simulink model "IMU_Simulation"  (Simulink 7.9)
settings: Solver=FixedStepDiscrete  StartTime=0.0  StopTime=25  FixedStep=.001  RelTol=1e-3
PreLoadFcn:
  | Script_Kalman
values from neighbouring files (symbols this model uses):
  Az = [1 -Ts ;0 1]    [Script_Kalman.m]
  Kz = 1e-3*[.4 ; -.04]    [Script_Kalman.m]
  Ts = .001    (= 0.001)    [Script_Kalman.m]
undefined symbols (not defined in the file or in its folder): dend, DiscIntNeverNeededParam, gaind, numd, polesd, zerosd
libraries: simulink x38
(part 2 of 2)

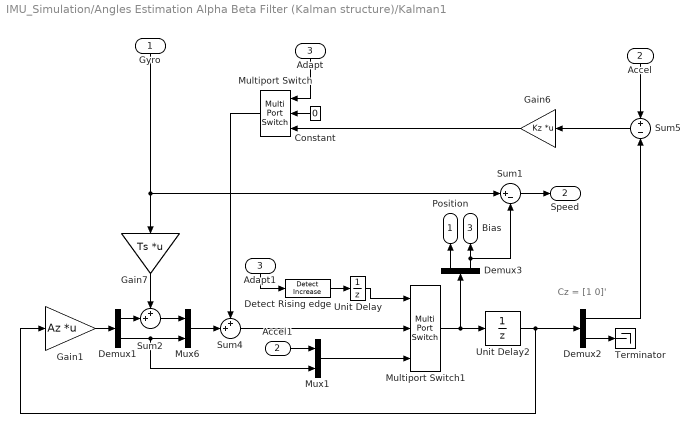
== system IMU_Simulation/Angles Estimation Alpha Beta Filter (Kalman structure)/Kalman1 ==
  note: Cz = [1 0]'
  Gyro : Inport
  Accel : Inport  Port=2
  Adapt : Inport  Port=3
  Accel1 : InportShadow  Port=2
  Adapt1 : InportShadow  Port=3
  Constant : Constant  Value=0
  Demux1 : Demux  Outputs=2
  Demux2 : Demux  Outputs=2
  Demux3 : Demux  Outputs=2
  Detect Rising edge : simulink/Logic and Bit Operations/Detect Increase  vinit=0  InputProcessing=Inherited  OutDataTypeStr=uint8
  Gain1 : Gain  Gain=Az  Multiplication=Matrix(K*u)
  Gain6 : Gain  Gain=Kz  Multiplication=Matrix(K*u)
  Gain7 : Gain  Gain=Ts  Multiplication=Matrix(K*u)
  Multiport Switch : MultiPortSwitch  DataPortOrder=Zero-based contiguous  Inputs=2  zeroidx=on
  Multiport Switch1 : MultiPortSwitch  DataPortOrder=Zero-based contiguous  Inputs=2  zeroidx=on
  Mux1 : Mux  Inputs=2
  Mux6 : Mux  Inputs=2
  Sum1 : Sum  Inputs=|+-
  Sum2 : Sum  Inputs=++|
  Sum4 : Sum  Inputs=++|
  Sum5 : Sum  Inputs=+-
  Terminator : Terminator
  Unit Delay : UnitDelay  SampleTime=-1
  Unit Delay2 : UnitDelay  SampleTime=-1
  Position : Outport
  Speed : Outport  Port=2
  Bias : Outport  Port=3
  wires:
  Sum1/1 -> Speed/1
  Demux3/2 -> Sum1/2, Bias/1
  Demux3/1 -> Position/1
  Unit Delay2/1 -> Gain1/1, Demux2/1
  Unit Delay/1 -> Multiport Switch1/1
  Gyro/1 -> Sum1/1, Gain7/1
  Accel/1 -> Sum5/1
  Gain7/1 -> Sum2/1
  Sum5/1 -> Gain6/1
  Mux6/1 -> Sum4/2
  Demux1/2 -> Mux6/2, Mux1/2
  Sum2/1 -> Mux6/1
  Demux1/1 -> Sum2/2
  Gain1/1 -> Demux1/1
  Demux2/1 -> Sum5/2
  Multiport Switch/1 -> Sum4/1
  Adapt/1 -> Multiport Switch/1
  Gain6/1 -> Multiport Switch/3
  Constant/1 -> Multiport Switch/2
  Detect Rising edge/1 -> Unit Delay/1
  Multiport Switch1/1 -> Demux3/1, Unit Delay2/1
  Sum4/1 -> Multiport Switch1/2
  Adapt1/1 -> Detect Rising edge/1
  Accel1/1 -> Mux1/1
  Mux1/1 -> Multiport Switch1/3
  Demux2/2 -> Terminator/1

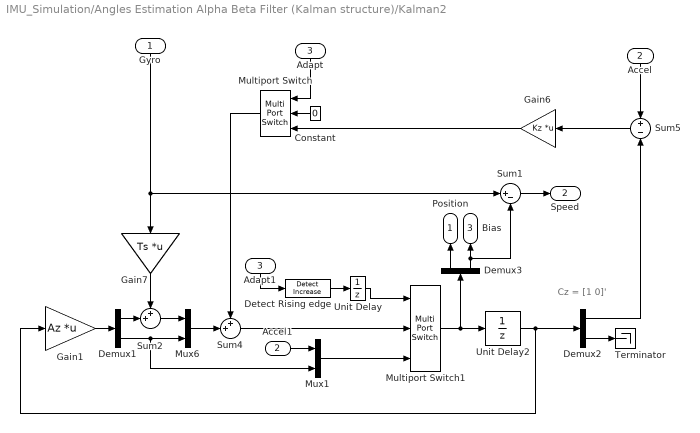
== system IMU_Simulation/Angles Estimation Alpha Beta Filter (Kalman structure)/Kalman2 ==
  note: Cz = [1 0]'
  Gyro : Inport
  Accel : Inport  Port=2
  Adapt : Inport  Port=3
  Accel1 : InportShadow  Port=2
  Adapt1 : InportShadow  Port=3
  Constant : Constant  Value=0
  Demux1 : Demux  Outputs=2
  Demux2 : Demux  Outputs=2
  Demux3 : Demux  Outputs=2
  Detect Rising edge : simulink/Logic and Bit Operations/Detect Increase  vinit=0  InputProcessing=Inherited  OutDataTypeStr=uint8
  Gain1 : Gain  Gain=Az  Multiplication=Matrix(K*u)
  Gain6 : Gain  Gain=Kz  Multiplication=Matrix(K*u)
  Gain7 : Gain  Gain=Ts  Multiplication=Matrix(K*u)
  Multiport Switch : MultiPortSwitch  DataPortOrder=Zero-based contiguous  Inputs=2  zeroidx=on
  Multiport Switch1 : MultiPortSwitch  DataPortOrder=Zero-based contiguous  Inputs=2  zeroidx=on
  Mux1 : Mux  Inputs=2
  Mux6 : Mux  Inputs=2
  Sum1 : Sum  Inputs=|+-
  Sum2 : Sum  Inputs=++|
  Sum4 : Sum  Inputs=++|
  Sum5 : Sum  Inputs=+-
  Terminator : Terminator
  Unit Delay : UnitDelay  SampleTime=-1
  Unit Delay2 : UnitDelay  SampleTime=-1
  Position : Outport
  Speed : Outport  Port=2
  Bias : Outport  Port=3
  wires:
  Demux2/2 -> Terminator/1
  Mux1/1 -> Multiport Switch1/3
  Accel1/1 -> Mux1/1
  Adapt1/1 -> Detect Rising edge/1
  Sum4/1 -> Multiport Switch1/2
  Multiport Switch1/1 -> Unit Delay2/1, Demux3/1
  Detect Rising edge/1 -> Unit Delay/1
  Constant/1 -> Multiport Switch/2
  Gain6/1 -> Multiport Switch/3
  Adapt/1 -> Multiport Switch/1
  Multiport Switch/1 -> Sum4/1
  Demux2/1 -> Sum5/2
  Gain1/1 -> Demux1/1
  Demux1/1 -> Sum2/2
  Sum2/1 -> Mux6/1
  Demux1/2 -> Mux1/2, Mux6/2
  Mux6/1 -> Sum4/2
  Sum5/1 -> Gain6/1
  Gain7/1 -> Sum2/1
  Accel/1 -> Sum5/1
  Gyro/1 -> Gain7/1, Sum1/1
  Unit Delay/1 -> Multiport Switch1/1
  Unit Delay2/1 -> Demux2/1, Gain1/1
  Demux3/1 -> Position/1
  Demux3/2 -> Bias/1, Sum1/2
  Sum1/1 -> Speed/1

== system IMU_Simulation/Angles Estimation Alpha Beta Filter (Kalman structure)/Norm L1 ==
  Accel Y : Inport
  Accel Z : Inport  Port=2
  Accel X : Inport  Port=3
  Abs : Abs
  Abs1 : Abs
  Abs2 : Abs
  Sum1 : Sum
  Sum3 : Sum
  abs(Y)+abs(Z) : Outport
  abs(X)+abs(Z) : Outport  Port=2
  wires:
  Abs/1 -> Sum3/1
  Abs1/1 -> Sum1/1, Sum3/2
  Accel Y/1 -> Abs/1
  Accel Z/1 -> Abs1/1
  Sum3/1 -> abs(Y)+abs(Z)/1
  Abs2/1 -> Sum1/2
  Accel X/1 -> Abs2/1
  Sum1/1 -> abs(X)+abs(Z)/1

== system IMU_Simulation/Angles Estimation Alpha Beta Filter (Kalman structure)/Simplified Kalman for publi ==
  note: Cz = [1 0]'
  Gyro : Inport
  Accel : Inport  Port=2
  Demux1 : Demux  Outputs=2
  Demux2 : Demux  Outputs=2
  Gain1 : Gain  Gain=Az  Multiplication=Matrix(K*u)
  Gain6 : Gain  Gain=Kz  Multiplication=Matrix(K*u)
  Gain7 : Gain  Gain=Ts  Multiplication=Matrix(K*u)
  Mux6 : Mux  Inputs=2
  Sum2 : Sum  Inputs=++|
  Sum4 : Sum  Inputs=++|
  Sum5 : Sum  Inputs=+-
  Terminator : Terminator
  Unit Delay2 : UnitDelay  SampleTime=-1
  Angle Estimation : Outport
  wires:
  Demux2/2 -> Terminator/1
  Sum4/1 -> Unit Delay2/1
  Demux2/1 -> Sum5/2, Angle Estimation/1
  Gain1/1 -> Demux1/1
  Demux1/1 -> Sum2/2
  Sum2/1 -> Mux6/1  "Angle Estimation"
  Demux1/2 -> Mux6/2  "Gyro Bias"
  Mux6/1 -> Sum4/2
  Sum5/1 -> Gain6/1
  Gain7/1 -> Sum2/1
  Accel/1 -> Sum5/1
  Gyro/1 -> Gain7/1
  Unit Delay2/1 -> Demux2/1, Gain1/1
  Gain6/1 -> Sum4/1

== system IMU_Simulation/Angles Estimation Alpha Beta Filter (Kalman structure)/Unwrap1 ==
  Estimated Angle : Inport
  Compare To Constant : simulink/Logic and Bit Operations/Compare To Constant  relop=>  const=180  OutDataTypeStr=uint8  ZeroCross=off
  Compare To Constant1 : simulink/Logic and Bit Operations/Compare To Constant  relop=<  const=-180  OutDataTypeStr=uint8  ZeroCross=off
  Compare To Zero : simulink/Logic and Bit Operations/Compare To Zero  relop=~=  OutDataTypeStr=uint8  ZeroCross=off
  Difference : simulink/Discrete/Difference  ICPrevInput=0.0  InputProcessing=Inherited  OutMin=[]  OutMax=[]  OutDataType=sfix(16)  OutScaling=2^-10  DoSatur=off
  Discrete-Time Integrator : DiscreteIntegrator  gainval=1000  SampleTime=-1  ICPrevOutput=DiscIntNeverNeededParam  ICPrevScaledInput=DiscIntNeverNeededParam
  Logical Operator : Logic  Operator=NOR  AllPortsSameDT=off  OutDataTypeStr=boolean
  Lookup Table : Lookup  InputValues=[-500 -195 195]  Table=[+360 0 -360]  LookUpMeth=Use Input Below
  Merge : Merge  Inputs=3
  Sum2 : Sum
  unwrap : Subsystem  TreatAsAtomicUnit=on
  unwrap1 : Subsystem  TreatAsAtomicUnit=on
  unwrap2 : Subsystem  TreatAsAtomicUnit=on
  unwrap angle : Outport
  Wrap : Outport  Port=2
  wires:
  Compare To Zero/1 -> Wrap/1
  Lookup Table/1 -> Compare To Zero/1, Sum2/1
  Merge/1 -> Sum2/2
  Sum2/1 -> Discrete-Time Integrator/1
  Difference/1 -> Compare To Constant/1, unwrap/1(In1), Compare To Constant1/1, unwrap1/1(In1), unwrap2/1(In1)
  Compare To Constant/1 -> Logical Operator/1, unwrap/Enable
  Compare To Constant1/1 -> unwrap1/Enable, Logical Operator/2
  Logical Operator/1 -> unwrap2/Enable
  unwrap2/1(Out1) -> Merge/1
  unwrap/1(Out1) -> Merge/2
  unwrap1/1(Out1) -> Merge/3
  Estimated Angle/1 -> Difference/1
  Discrete-Time Integrator/1 -> Lookup Table/1, unwrap angle/1

== system IMU_Simulation/Angles Estimation Alpha Beta Filter (Kalman structure)/Unwrap2 ==
  Estimated Angle : Inport
  Compare To Constant : simulink/Logic and Bit Operations/Compare To Constant  relop=>  const=180  OutDataTypeStr=uint8  ZeroCross=off
  Compare To Constant1 : simulink/Logic and Bit Operations/Compare To Constant  relop=<  const=-180  OutDataTypeStr=uint8  ZeroCross=off
  Compare To Zero : simulink/Logic and Bit Operations/Compare To Zero  relop=~=  OutDataTypeStr=uint8  ZeroCross=off
  Difference : simulink/Discrete/Difference  ICPrevInput=0.0  InputProcessing=Inherited  OutMin=[]  OutMax=[]  OutDataType=sfix(16)  OutScaling=2^-10  DoSatur=off
  Discrete-Time Integrator : DiscreteIntegrator  gainval=1000  SampleTime=-1  ICPrevOutput=DiscIntNeverNeededParam  ICPrevScaledInput=DiscIntNeverNeededParam
  Logical Operator : Logic  Operator=NOR  AllPortsSameDT=off  OutDataTypeStr=boolean
  Lookup Table : Lookup  InputValues=[-500 -195 195]  Table=[+360 0 -360]  LookUpMeth=Use Input Below
  Merge : Merge  Inputs=3
  Sum2 : Sum
  unwrap : Subsystem  TreatAsAtomicUnit=on
  unwrap1 : Subsystem  TreatAsAtomicUnit=on
  unwrap2 : Subsystem  TreatAsAtomicUnit=on
  unwrap angle : Outport
  Wrap : Outport  Port=2
  wires:
  Discrete-Time Integrator/1 -> unwrap angle/1, Lookup Table/1
  Estimated Angle/1 -> Difference/1
  unwrap1/1(Out1) -> Merge/3
  unwrap/1(Out1) -> Merge/2
  unwrap2/1(Out1) -> Merge/1
  Logical Operator/1 -> unwrap2/Enable
  Compare To Constant1/1 -> Logical Operator/2, unwrap1/Enable
  Compare To Constant/1 -> unwrap/Enable, Logical Operator/1
  Difference/1 -> unwrap2/1(In1), unwrap1/1(In1), Compare To Constant1/1, unwrap/1(In1), Compare To Constant/1
  Sum2/1 -> Discrete-Time Integrator/1
  Merge/1 -> Sum2/2
  Lookup Table/1 -> Sum2/1, Compare To Zero/1
  Compare To Zero/1 -> Wrap/1

== system IMU_Simulation/Angle Estimation Complementary Filter Order 1/Unwrap1/unwrap ==
  In1 : Inport
  Enable : EnablePort
  Bias2 : Constant  Value=-360
  Sum2 : Sum
  Out1 : Outport
  wires:
  Bias2/1 -> Sum2/2
  Sum2/1 -> Out1/1
  In1/1 -> Sum2/1

== system IMU_Simulation/Angle Estimation Complementary Filter Order 1/Unwrap1/unwrap1 ==
  In1 : Inport
  Enable : EnablePort
  Bias2 : Constant  Value=360
  Sum2 : Sum
  Out1 : Outport
  wires:
  Sum2/1 -> Out1/1
  Bias2/1 -> Sum2/2
  In1/1 -> Sum2/1

== system IMU_Simulation/Angle Estimation Complementary Filter Order 1/Unwrap1/unwrap2 ==
  In1 : Inport
  Enable : EnablePort
  Out1 : Outport
  wires:
  In1/1 -> Out1/1

== system IMU_Simulation/Angle Estimation Complementary Filter Order 1/Unwrap2/unwrap ==
  In1 : Inport
  Enable : EnablePort
  Bias2 : Constant  Value=-360
  Sum2 : Sum
  Out1 : Outport
  wires:
  In1/1 -> Sum2/1
  Sum2/1 -> Out1/1
  Bias2/1 -> Sum2/2

== system IMU_Simulation/Angle Estimation Complementary Filter Order 1/Unwrap2/unwrap1 ==
  In1 : Inport
  Enable : EnablePort
  Bias2 : Constant  Value=360
  Sum2 : Sum
  Out1 : Outport
  wires:
  In1/1 -> Sum2/1
  Bias2/1 -> Sum2/2
  Sum2/1 -> Out1/1

== system IMU_Simulation/Angle Estimation Complementary Filter Order 1/Unwrap2/unwrap2 ==
  In1 : Inport
  Enable : EnablePort
  Out1 : Outport
  wires:
  In1/1 -> Out1/1

== system IMU_Simulation/Angle Estimation Complementary Filter Order 2/Unwrap1/unwrap ==
  In1 : Inport
  Enable : EnablePort
  Bias2 : Constant  Value=-360
  Sum2 : Sum
  Out1 : Outport
  wires:
  In1/1 -> Sum2/1
  Sum2/1 -> Out1/1
  Bias2/1 -> Sum2/2

== system IMU_Simulation/Angle Estimation Complementary Filter Order 2/Unwrap1/unwrap1 ==
  In1 : Inport
  Enable : EnablePort
  Bias2 : Constant  Value=360
  Sum2 : Sum
  Out1 : Outport
  wires:
  In1/1 -> Sum2/1
  Bias2/1 -> Sum2/2
  Sum2/1 -> Out1/1

== system IMU_Simulation/Angle Estimation Complementary Filter Order 2/Unwrap1/unwrap2 ==
  In1 : Inport
  Enable : EnablePort
  Out1 : Outport
  wires:
  In1/1 -> Out1/1

== system IMU_Simulation/Angle Estimation Complementary Filter Order 2/Unwrap2/unwrap ==
  In1 : Inport
  Enable : EnablePort
  Bias2 : Constant  Value=-360
  Sum2 : Sum
  Out1 : Outport
  wires:
  Bias2/1 -> Sum2/2
  Sum2/1 -> Out1/1
  In1/1 -> Sum2/1

== system IMU_Simulation/Angle Estimation Complementary Filter Order 2/Unwrap2/unwrap1 ==
  In1 : Inport
  Enable : EnablePort
  Bias2 : Constant  Value=360
  Sum2 : Sum
  Out1 : Outport
  wires:
  Sum2/1 -> Out1/1
  Bias2/1 -> Sum2/2
  In1/1 -> Sum2/1

== system IMU_Simulation/Angle Estimation Complementary Filter Order 2/Unwrap2/unwrap2 ==
  In1 : Inport
  Enable : EnablePort
  Out1 : Outport
  wires:
  In1/1 -> Out1/1

== system IMU_Simulation/Angles Estimation (Ref: Pisano 2005)/Pisano/Low Pass1 ==
  In1 : Inport
  Discrete Zero-Pole : DiscreteZeroPole  Zeros=zerosd  Poles=polesd  Gain=gaind  SampleTime=SampleTime
  Out1 : Outport
  wires:
  Discrete Zero-Pole/1 -> Out1/1
  In1/1 -> Discrete Zero-Pole/1

== system IMU_Simulation/Angles Estimation (Ref: Pisano 2005)/Pisano1/Low Pass1 ==
  In1 : Inport
  Discrete Zero-Pole : DiscreteZeroPole  Zeros=zerosd  Poles=polesd  Gain=gaind  SampleTime=SampleTime
  Out1 : Outport
  wires:
  In1/1 -> Discrete Zero-Pole/1
  Discrete Zero-Pole/1 -> Out1/1

== system IMU_Simulation/Angles Estimation (Ref: Pisano 2005)/Unwrap1/unwrap ==
  In1 : Inport
  Enable : EnablePort
  Bias2 : Constant  Value=-360
  Sum2 : Sum
  Out1 : Outport
  wires:
  Bias2/1 -> Sum2/2
  Sum2/1 -> Out1/1
  In1/1 -> Sum2/1

== system IMU_Simulation/Angles Estimation (Ref: Pisano 2005)/Unwrap1/unwrap1 ==
  In1 : Inport
  Enable : EnablePort
  Bias2 : Constant  Value=360
  Sum2 : Sum
  Out1 : Outport
  wires:
  Sum2/1 -> Out1/1
  Bias2/1 -> Sum2/2
  In1/1 -> Sum2/1

== system IMU_Simulation/Angles Estimation (Ref: Pisano 2005)/Unwrap1/unwrap2 ==
  In1 : Inport
  Enable : EnablePort
  Out1 : Outport
  wires:
  In1/1 -> Out1/1

== system IMU_Simulation/Angles Estimation (Ref: Pisano 2005)/Unwrap2/unwrap ==
  In1 : Inport
  Enable : EnablePort
  Bias2 : Constant  Value=-360
  Sum2 : Sum
  Out1 : Outport
  wires:
  In1/1 -> Sum2/1
  Sum2/1 -> Out1/1
  Bias2/1 -> Sum2/2

== system IMU_Simulation/Angles Estimation (Ref: Pisano 2005)/Unwrap2/unwrap1 ==
  In1 : Inport
  Enable : EnablePort
  Bias2 : Constant  Value=360
  Sum2 : Sum
  Out1 : Outport
  wires:
  In1/1 -> Sum2/1
  Bias2/1 -> Sum2/2
  Sum2/1 -> Out1/1

== system IMU_Simulation/Angles Estimation (Ref: Pisano 2005)/Unwrap2/unwrap2 ==
  In1 : Inport
  Enable : EnablePort
  Out1 : Outport
  wires:
  In1/1 -> Out1/1

== system IMU_Simulation/Angles Estimation Alpha Beta Filter (Kalman structure)/Unwrap1/unwrap ==
  In1 : Inport
  Enable : EnablePort
  Bias2 : Constant  Value=-360
  Sum2 : Sum
  Out1 : Outport
  wires:
  In1/1 -> Sum2/1
  Sum2/1 -> Out1/1
  Bias2/1 -> Sum2/2

== system IMU_Simulation/Angles Estimation Alpha Beta Filter (Kalman structure)/Unwrap1/unwrap1 ==
  In1 : Inport
  Enable : EnablePort
  Bias2 : Constant  Value=360
  Sum2 : Sum
  Out1 : Outport
  wires:
  In1/1 -> Sum2/1
  Bias2/1 -> Sum2/2
  Sum2/1 -> Out1/1

== system IMU_Simulation/Angles Estimation Alpha Beta Filter (Kalman structure)/Unwrap1/unwrap2 ==
  In1 : Inport
  Enable : EnablePort
  Out1 : Outport
  wires:
  In1/1 -> Out1/1

== system IMU_Simulation/Angles Estimation Alpha Beta Filter (Kalman structure)/Unwrap2/unwrap ==
  In1 : Inport
  Enable : EnablePort
  Bias2 : Constant  Value=-360
  Sum2 : Sum
  Out1 : Outport
  wires:
  Bias2/1 -> Sum2/2
  Sum2/1 -> Out1/1
  In1/1 -> Sum2/1

== system IMU_Simulation/Angles Estimation Alpha Beta Filter (Kalman structure)/Unwrap2/unwrap1 ==
  In1 : Inport
  Enable : EnablePort
  Bias2 : Constant  Value=360
  Sum2 : Sum
  Out1 : Outport
  wires:
  Sum2/1 -> Out1/1
  Bias2/1 -> Sum2/2
  In1/1 -> Sum2/1

== system IMU_Simulation/Angles Estimation Alpha Beta Filter (Kalman structure)/Unwrap2/unwrap2 ==
  In1 : Inport
  Enable : EnablePort
  Out1 : Outport
  wires:
  In1/1 -> Out1/1
